simulink model "HNDF2"  (R2023b)
settings: Solver=FixedStepAuto  StartTime=0.0  StopTime=1  FixedStep=2*NN/Fs  RelTol=1e-3
undefined symbols (not defined in the file or in its folder): A2, AA2, Fs, NN
settings Model: Creator=mpolj  LastModifiedBy=mpolj

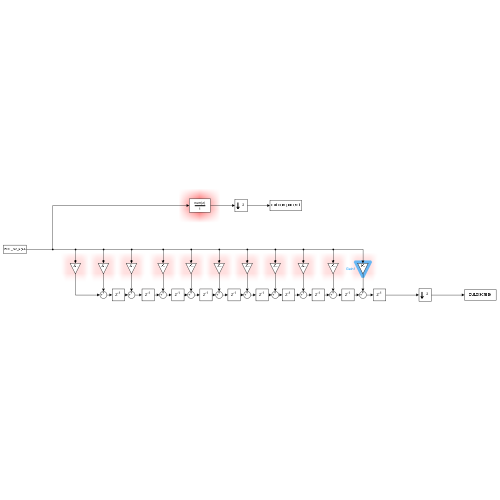
[thumbnail: Simulink's stored preview of the top-level diagram]
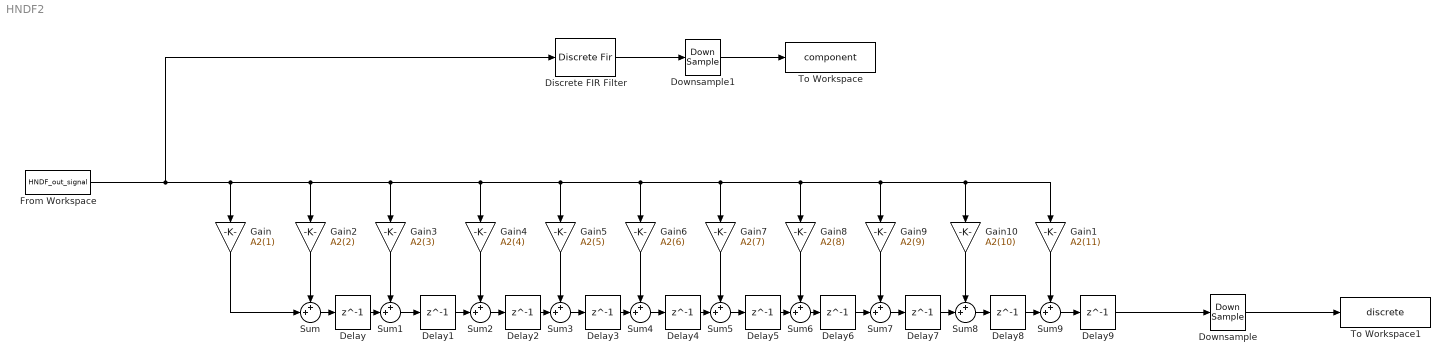
== system HNDF2 ==
  Delay{,1..9} (10 alike) : Delay  DelayLength=1  InitialCondition=0
  Discrete FIR Filter : DiscreteFir  Coefficients=AA2
  Downsample : DownSample  AllowArbitraryFixedInput=on
  Downsample1 : DownSample  AllowArbitraryFixedInput=on
  From Workspace : FromWorkspace  VariableName=HNDF_out_signal
  Gain : Gain  Gain=A2(1)
  Gain1 : Gain  Gain=A2(11)
  Gain10 : Gain  Gain=A2(10)
  Gain2 : Gain  Gain=A2(2)
  Gain3 : Gain  Gain=A2(3)
  Gain4 : Gain  Gain=A2(4)
  Gain5 : Gain  Gain=A2(5)
  Gain6 : Gain  Gain=A2(6)
  Gain7 : Gain  Gain=A2(7)
  Gain8 : Gain  Gain=A2(8)
  Gain9 : Gain  Gain=A2(9)
  Sum{,1..9} (10 alike) : Sum  Inputs=++|
  To Workspace : ToWorkspace  VariableName=component  SaveFormat=Timeseries  SampleTime=4*NN/Fs
  To Workspace1 : ToWorkspace  VariableName=discrete  SaveFormat=Timeseries  SampleTime=4*NN/Fs
  wires:
  Discrete FIR Filter/1 -> Downsample1/1
  Sum/1 -> Delay/1
  Gain2/1 -> Sum/1
  Gain/1 -> Sum/2
  Sum1/1 -> Delay1/1
  Gain3/1 -> Sum1/1
  Delay/1 -> Sum1/2
  From Workspace/1 -> Discrete FIR Filter/1, Gain/1, Gain2/1, Gain3/1, Gain4/1, Gain5/1, Gain6/1, Gain7/1, Gain8/1, Gain9/1, Gain1/1, Gain10/1
  Delay2/1 -> Sum3/2
  Sum3/1 -> Delay3/1
  Gain5/1 -> Sum3/1
  Sum2/1 -> Delay2/1
  Gain4/1 -> Sum2/1
  Delay1/1 -> Sum2/2
  Delay4/1 -> Sum5/2
  Sum5/1 -> Delay5/1
  Gain7/1 -> Sum5/1
  Sum4/1 -> Delay4/1
  Gain6/1 -> Sum4/1
  Delay6/1 -> Sum7/2
  Sum7/1 -> Delay7/1
  Gain9/1 -> Sum7/1
  Sum6/1 -> Delay6/1
  Gain8/1 -> Sum6/1
  Delay8/1 -> Sum9/2
  Sum9/1 -> Delay9/1
  Gain1/1 -> Sum9/1
  Sum8/1 -> Delay8/1
  Gain10/1 -> Sum8/1
  Delay3/1 -> Sum4/2
  Delay5/1 -> Sum6/2
  Delay7/1 -> Sum8/2
  Delay9/1 -> Downsample/1
  Downsample/1 -> To Workspace1/1
  Downsample1/1 -> To Workspace/1
